simulink model "stateMonitor"  (R2025b)
settings: Solver=FixedStepAuto  StartTime=0.0  StopTime=10.0  FixedStep=0.5  RelTol=1e-3
PreLoadFcn:
  | stepsize_mon = evalin('base', get_param(bdroot, 'FixedStep'));
  | 
  | if(~exist('t_end','var'))
  |     t_end = 0; %Placeholder for HiL
  | end
undefined symbols (not defined in the file or in its folder): defaultConsts
settings Model: Creator=ac124458  LastModifiedBy=ac124458
settings SolverCC: AlgebraicLoopSolver=TrustRegion
settings DebuggingCC: UnconnectedInputMsg=warning  UnconnectedOutputMsg=warning  UnconnectedLineMsg=warning
settings ModelReferenceCC: EnableRefExpFcnMdlSchedulingChecks=on
settings RTWCC: GPUComputeCapability=3.5

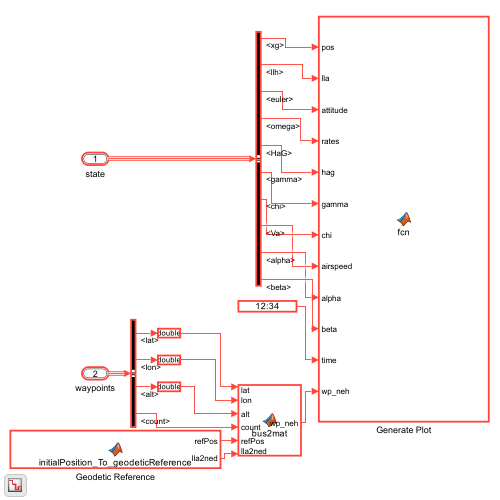
[thumbnail: Simulink's stored preview of the top-level diagram]
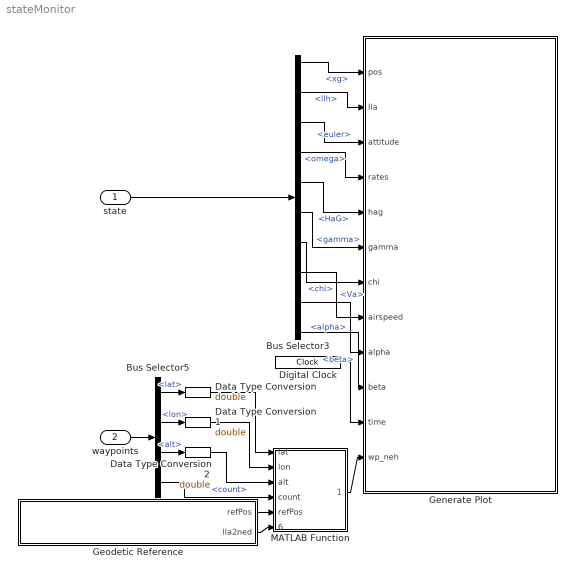
== system stateMonitor ==
  state : Inport  OutDataTypeStr=Bus: fmBus
  waypoints : Inport  Port=2  OutDataTypeStr=Bus: waypoint_list_bus
  Bus Selector3 : BusSelector  OutputSignals=rigidbodyBus.xg,rigidbodyBus.llh,rigidbodyBus.euler,rigidbodyBus.omega,utilityBus.HaG,rigidbodyBus.gamma,rigidbodyBus.chi,atmosBus.Va,atmosBus.alpha,atmosBus.beta
  Bus Selector5 : BusSelector  OutputSignals=lat,lon,alt,count
  Data Type Conversion : DataTypeConversion  OutDataTypeStr=double  SaturateOnIntegerOverflow=off  RndMeth=Floor
  Data Type Conversion1 : DataTypeConversion  OutDataTypeStr=double  SaturateOnIntegerOverflow=off  RndMeth=Floor
  Data Type Conversion2 : DataTypeConversion  OutDataTypeStr=double  SaturateOnIntegerOverflow=off  RndMeth=Floor
  Digital Clock : DigitalClock  SampleTime=stepsize_mon
  Generate Plot : MATLAB Function  TreatAsAtomicUnit=on
  Geodetic Reference : MATLAB Function  TreatAsAtomicUnit=on
  MATLAB Function : MATLAB Function  TreatAsAtomicUnit=on
  wires:
  Bus Selector3/5 -> Generate Plot/5(hag)  "<HaG>"
  Bus Selector3/4 -> Generate Plot/4(rates)  "<omega>"
  Bus Selector3/9 -> Generate Plot/9(alpha)  "<alpha>"
  Bus Selector3/7 -> Generate Plot/7(chi)  "<chi>"
  Bus Selector3/8 -> Generate Plot/8(airspeed)  "<Va>"
  MATLAB Function/1(wp_neh) -> Generate Plot/12(wp_neh)
  Bus Selector3/6 -> Generate Plot/6(gamma)  "<gamma>"
  Bus Selector3/3 -> Generate Plot/3(attitude)  "<euler>"
  Bus Selector3/1 -> Generate Plot/1(pos)  "<xg>"
  Bus Selector3/10 -> Generate Plot/10(beta)  "<beta>"
  Bus Selector3/2 -> Generate Plot/2(lla)  "<llh>"
  Digital Clock/1 -> Generate Plot/11(time)
  state/1 -> Bus Selector3/1
  Geodetic Reference/2(lla2ned) -> MATLAB Function/6(lla2ned)
  Geodetic Reference/1(refPos) -> MATLAB Function/5(refPos)
  waypoints/1 -> Bus Selector5/1
  Bus Selector5/1 -> Data Type Conversion/1  "<lat>"
  Bus Selector5/2 -> Data Type Conversion1/1  "<lon>"
  Bus Selector5/3 -> Data Type Conversion2/1  "<alt>"
  Bus Selector5/4 -> MATLAB Function/4(count)  "<count>"
  Data Type Conversion/1 -> MATLAB Function/1(lat)
  Data Type Conversion1/1 -> MATLAB Function/2(lon)
  Data Type Conversion2/1 -> MATLAB Function/3(alt)

== matlab function stateMonitor/Generate Plot ==
  data: pos input; lla input; attitude input; rates input; hag input; gamma input; chi input; airspeed input; alpha input; beta input; time input; wp_neh input; t_end parameter; defaultConsts parameter
function fcn(pos,lla,attitude,rates,hag,gamma,chi,airspeed,alpha,beta,time,wp_neh,t_end,defaultConsts)
coder.extrinsic('delete');

pos(3) = -lla(3);

% coder.extrinsic('plot')
coder.extrinsic('animatedline')
coder.extrinsic('addpoints')
coder.extrinsic('clearpoints')
coder.extrinsic('get_param')

persistent fig
persistent handleWP handlePos handlePhi handleTheta handlePsi handleP handleQ handleR handleHaG handleGamma handleChi handleVA handleAlpha handleBeta;

if t_end<=0
    time_window = [max(0,time-50),time+20];
else
    time_window = [0,t_end];
end

if isempty(fig)
    
    close all
    fig = figure('Name','State Monitor','WindowStyle','docked');
    
    subplot(10,2,[1,2,3,4,5,6,7,8])
    
    hold on
    handleWP = animatedline(0,0,defaultConsts.initialPositionLla(3),'Color','k','LineStyle','--','Marker','x');
    handlePos = animatedline(0,0,defaultConsts.initialPositionLla(3),'Color','r','LineWidth',1.5);
    clearpoints(handlePos)
    
    xlabel('East [m]');
    ylabel('North [m]');
    zlabel('Height [m]');
    ground = -defaultConsts.initialPositionLla(3);
    axis([-350 600 -700 200 -ground -ground+200])
    view(83,11)
    axis equal
    grid on;
    
    subplot(10,2,9)
    handlePhi = animatedline(0,0,'Color','r','LineWidth',1.5);
    xlim(time_window);
    ylim([-50,50]);
    ylabel('$\phi \; [^\circ]$','Interpreter','latex');
    grid on;
    
    subplot(10,2,11)
    handleTheta = animatedline(0,0,'Color','r','LineWidth',1.5);
    xlim(time_window);
    ylim([-15,15]);
    ylabel('$\theta \; [^\circ]$','Interpreter','latex');
    grid on;
    
    subplot(10,2,13)
    handlePsi = animatedline(0,0,'Color','r','LineWidth',1.5);
    xlim(time_window);
    ylim([-180,180]);
    ylabel('$\psi \; [^\circ]$','Interpreter','latex');
    grid on;
    
    subplot(10,2,10)
    handleHaG = animatedline(0,0,'Color','r','LineWidth',1.5);
    xlim(time_window);
    ylim([0,50]);
    ylabel('$HaG$ [m]','Interpreter','latex');
    grid on;
    
    subplot(10,2,12)
    handleGamma = animatedline(0,0,'Color','r','LineWidth',1.5);
    xlim(time_window);
    ylim([-15,15]);
    ylabel('$\gamma \; [^\circ]$','Interpreter','latex');
    grid on;
    
    subplot(10,2,14)
    handleChi = animatedline(0,0,'Color','r','LineWidth',1.5);
    xlim(time_window);
    ylim([-180,180]);
    ylabel('$\chi \; [^\circ]$','Interpreter','latex');
    grid on;
    
    subplot(10,2,15)
    handleP = animatedline(0,0,'Color','r','LineWidth',1.5);
    xlim(time_window);
    ylim([-60,60]);
    ylabel('$p \; [^\circ$/s]','Interpreter','latex');
    grid on;
    
    subplot(10,2,17)
    handleQ = animatedline(0,0,'Color','r','LineWidth',1.5);
    xlim(time_window);
    ylim([-60,60]);
    ylabel('$q \; [^\circ]$','Interpreter','latex');
    grid on;
    
    subplot(10,2,19)
    handleR = animatedline(0,0,'Color','r','LineWidth',1.5);
    xlim(time_window);
    ylim([-60,60]);
    ylabel('$r \; [^\circ]$','Interpreter','latex');
    xlabel('Time [s]');
    grid on;
    
    subplot(10,2,16)
    handleVA = animatedline(0,0,'Color','r','LineWidth',1.5);
    xlim(time_window);
    ylim([0,30]);
    ylabel('$V_A$ [m/s]','Interpreter','latex');
    grid on;
    
    subplot(10,2,18)
    handleAlpha = animatedline(0,0,'Color','r','LineWidth',1.5);
    xlim(time_window);
    ylim([-15,15]);
    ylabel('$\alpha \; [^\circ]$','Interpreter','latex');
    grid on;
    
    subplot(10,2,20)
    handleBeta = animatedline(0,0,'Color','r','LineWidth',1.5);
    xlim(time_window);
    ylim([-20,20]);
    ylabel('$\beta \; [^\circ]$','Interpreter','latex');
    xlabel('Time [s]');
    grid on;
end

%Waypoints
wp_neh = double(wp_neh);
wp_count = min(wp_neh(1,1),20);
clearpoints(handleWP)
delete(findobj(gcf,'type','text'));

if wp_count>=1
    for i=2:(wp_count+1)
        addpoints(handleWP, wp_neh(i,2), wp_neh(i,1), -wp_neh(i,3));
        text(wp_neh(i,2), wp_neh(i,1), -wp_neh(i,3)-10, int2str(i-1));
    end
    addpoints(handleWP, wp_neh(2,2), wp_neh(2,1), -wp_neh(2,3)); %back to first wp
end

%Current position
addpoints(handlePos,pos(2),pos(1),-pos(3));

%Graphs
addpoints(handlePhi,time,rad2deg(attitude(1)));
addpoints(handleTheta,time,rad2deg(attitude(2)));
addpoints(handlePsi,time,rad2deg(attitude(3)));

addpoints(handleP,time,rad2deg(rates(1)));
addpoints(handleQ,time,rad2deg(rates(2)));
addpoints(handleR,time,rad2deg(rates(3)));

addpoints(handleHaG,time,hag);
addpoints(handleGamma,time,rad2deg(gamma));
addpoints(handleChi,time,rad2deg(chi));

addpoints(handleVA,time,airspeed);
addpoints(handleAlpha,time,rad2deg(alpha));
addpoints(handleBeta,time,rad2deg(beta));

drawnow limitrate

end

== matlab function stateMonitor/MATLAB Function ==
  data: lat input double size=20; lon input double size=20; alt input double size=20; count input uint16; refPos input; lla2ned input; wp_neh output size=[21,3]
function wp_neh = bus2mat(lat,lon,alt,count,refPos,lla2ned)
NUM_WP = length(lat);

persistent waypoints_stored_lat waypoints_stored_lon waypoints_stored_alt waypoints_stored_count

if (isempty(waypoints_stored_lat) || isempty(waypoints_stored_lon) || isempty(waypoints_stored_alt) || isempty(waypoints_stored_count))
    waypoints_stored_lat = zeros(NUM_WP);
    waypoints_stored_lon = zeros(NUM_WP);
    waypoints_stored_alt = zeros(NUM_WP);
    waypoints_stored_count = single(0);
end

if (lat(1) && count<NUM_WP+1 && (count)>0)
    waypoints_stored_lat = lat;
    waypoints_stored_lon = lon;
    waypoints_stored_alt = alt;
    waypoints_stored_count = single(count);
end

temp_LlaRawToNed = single([0.011; 0.007; 0.001]);
temp_PosLlaRaw = single([487396608.0; 89221688.0; 483623.0]);

if ((refPos(1)))
    temp_PosLlaRaw = single(refPos);
    temp_LlaRawToNed = lla2ned;
end

wp_neh = zeros(NUM_WP+1, 3, 'single');
if (((waypoints_stored_count) > 0) && ((waypoints_stored_count) < NUM_WP+1))
    wp_neh(1, 1) = single(waypoints_stored_count);
    for i=2:(waypoints_stored_count+1)
        coordsLlu = [waypoints_stored_lat(i-1)*1e7, waypoints_stored_lon(i-1)*1e7, waypoints_stored_alt(i-1)*1e3];
        coordsNED = temp_LlaRawToNed(1:2).*(single(coordsLlu(1:2)')-temp_PosLlaRaw(1:2));
        wp_neh(i, 1) = coordsNED(1);
        wp_neh(i, 2) = coordsNED(2);
        wp_neh(i, 3) = temp_LlaRawToNed(3).*(single(coordsLlu(3)')+temp_PosLlaRaw(3));
    end
end
end

== matlab function stateMonitor/Geodetic Reference ==
  settings: updateMethod=DISCRETE
  data: refPos output; defaultConsts parameter size=1; lla2ned output
function [refPos,lla2ned]  =initialPosition_To_geodeticReference(defaultConsts)
persistent refPosLlhRaw refLlhRawToNed
if isempty(refPosLlhRaw)
    semiMajorAxis=single(6378137);
    eccentricity=single(8.1819190842622e-2);
    posScaleFactor=single([1e-7*pi/180; 1e-7*pi/180; 1e-3]);
    
    refPosLlhRaw = int32([defaultConsts.initialPositionLla(1:2)*1e7; defaultConsts.initialPositionLla(3)*1e3]);
    R0=semiMajorAxis/sqrt(1-eccentricity^2*sin(posScaleFactor(1)*single(refPosLlhRaw(1)))^2);
    refLlhRawToNed = [(1-eccentricity^2)/semiMajorAxis^2*R0^3+posScaleFactor(3)*single(refPosLlhRaw(3)); (R0+posScaleFactor(3)*single(refPosLlhRaw(3)))*cos(posScaleFactor(1)*single(refPosLlhRaw(1))); -1].*posScaleFactor;
end
refPos = refPosLlhRaw;
lla2ned = refLlhRawToNed;
end
